simulink model "Battery_droop_control_4"  (R2022a)
settings: Solver=ode23tb  StartTime=0.0  StopTime=1  RelTol=1e-3  EnableMultiTasking=on
values from neighbouring files (symbols this model uses):
  R_power_mode_load_change = zeros(1, length(load_percent_list))    [Battery_charge_discharge_FSBB_param_init.m]
  R_voltage_mode_load_change = zeros(1, length(load_percent_list))    [Battery_charge_discharge_FSBB_param_init.m]
  time_step = 1 / wave_freq    (= 2.22222222222e-05)    [Battery_charge_discharge_FSBB_param_init.m]
undefined symbols (not defined in the file or in its folder): Ion, Lithium
libraries: spsSeriesRLCBranchLib x27, spsTriangleGeneratorLib x16, slpidlib x14, spsCurrentMeasurementLib x9, spsIGBTDiodeLib x8, spsIdealSwitchLib x8, spsVoltageMeasurementLib x8, simulink x4, spsBatteryLib x3, spsControlledVoltageSourceLib x3, eeGeneralControl x2, spspowerguiLib x1
(part 3 of 4)

== system Battery_droop_control_4/InitSystem ==

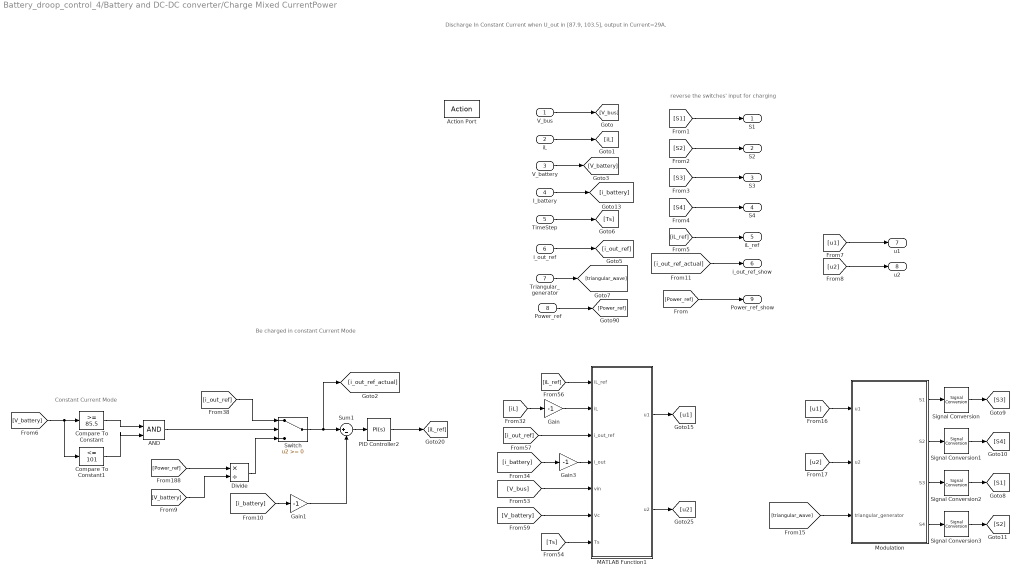
== system Battery_droop_control_4/Battery and DC-DC converter/Charge Mixed CurrentPower ==
  note: Discharge In Constant Current
      | when U_out in [87.9, 103.5], output in Current=29A.
  note: reverse the switches' input for charging
  note: Be charged in constant Current Mode
  note: Constant Current Mode
  V_bus : Inport
  iL : Inport  Port=2
  V_battery : Inport  Port=3
  I_battery : Inport  Port=4
  TimeStep : Inport  Port=5
  i_out_ref : Inport  Port=6
  Triangular_generator : Inport  Port=7
  Power_ref : Inport  Port=8
  Action Port : ActionPort  ActionPortLabel=elseif(u1 == 0 & (u3>=85.5 & u3 <= 116.15))
  AND : Logic  IconShape=distinctive  AllPortsSameDT=off  OutDataTypeStr=boolean
  Compare To Constant : simulink/Logic and Bit Operations/Compare To Constant  relop=>=  const=85.5  OutDataTypeStr=boolean
  Compare To Constant1 : simulink/Logic and Bit Operations/Compare To Constant  relop=<=  const=101  OutDataTypeStr=boolean
  Divide : Product  Inputs=*/
  Gain : Gain  Gain=-1
  Gain1 : Gain  Gain=-1
  Gain3 : Gain  Gain=-1
  MATLAB Function1 : MATLAB Function  TreatAsAtomicUnit=on
  Modulation : Subsystem
  PID Controller2 : slpidlib/PID Controller  Controller=PI  Form=Parallel  TimeDomain=Continuous-time  UseExternalTs=off  SampleTime=-1  IntegratorMethod=Forward Euler  FilterMethod=Forward Euler  ControllerParametersSource=internal  P=15/3  I=1000  UseKiTs=on  D=0  N=100  UseFilter=on  TunerSelectOption=Transfer Function Based (PID Tuner App)  InitialConditionSource=internal  InitialConditionForIntegrator=0  InitialConditionForFilter=0  DifferentiatorICPrevScaledInput=0  ExternalReset=none  TrackingMode=off  Kt=1  LimitOutput=on  SatLimitsSource=internal  UpperSaturationLimit=50  LowerSaturationLimit=-10  LinearizeAsGain=on  AntiWindupMode=clamping  Kb=1  POutMin=[]  POutMax=[]  IOutMin=[]  IOutMax=[]  DOutMin=[]  DOutMax=[]  NOutMin=[]  NOutMax=[]  SumOutMin=[]  SumOutMax=[]  SaturationOutMin=[]  SaturationOutMax=[]  PParamMin=[]  PParamMax=[]  IParamMin=[]  IParamMax=[]  DParamMin=[]  DParamMax=[]  NParamMin=[]  NParamMax=[]  KbParamMin=[]  KbParamMax=[]  KtParamMin=[]  KtParamMax=[]  KbOutMin=[]  KbOutMax=[]  KtOutMin=[]  KtOutMax=[]  IntegratorOutMin=[]  IntegratorOutMax=[]  FilterOutMin=[]  FilterOutMax=[]  SumI1OutMin=[]  SumI1OutMax=[]  SumI2OutMin=[]  SumI2OutMax=[]  SumI3OutMin=[]  SumI3OutMax=[]  SumI4OutMin=[]  SumI4OutMax=[]  SumDOutMin=[]  SumDOutMax=[]  DifferentiatorOutMin=[]  DifferentiatorOutMax=[]  FilterDiffOutCoefMin=[]  FilterDiffOutCoefMax=[]  ReciprocalOutMin=[]  ReciprocalOutMax=[]  SumDenOutMin=[]  SumDenOutMax=[]  SumNumOutMin=[]  SumNumOutMax=[]  DivideOutMin=[]  DivideOutMax=[]  UdiffTsProdOutMin=[]  UdiffTsProdOutMax=[]  NTsProdOutMin=[]  NTsProdOutMax=[]  UintegralTsProdOutMin=[]  UintegralTsProdOutMax=[]  UngainTsProdOutMin=[]  UngainTsProdOutMax=[]  IntegratorContinuousStateAttributes=''  IntegratorStateMustResolveToSignalObject=off  IntegratorRTWStateStorageClass=Auto  FilterContinuousStateAttributes=''  FilterStateMustResolveToSignalObject=off  FilterRTWStateStorageClass=Auto  ParallelPVariant=InternalParameters  IdealPVariant=Disabled  IVariant=InternalParameters  DVariant=Disabled  IntegratorVariant=Continuous  SatVariant=Enabled  AWVariant=ContClampingParallel  PCopyVariant=Disabled  TRVariant=Disabled  FdbkBlocksVariant=Forward  IdealPFdbkVariant=Disabled  SatFdbkVariant=Disabled  DerivativeFilterVariant=Disabled  NVariant=Disabled  NCopyVariant=Disabled_SignalSpec  FilterICVariant=Disabled  IntegratorICVariant=InternalICs  ExternalResetVariant=Disabled  TRSumVariant=Passthrough  SumFdbkVariant=Disabled  SumVariant=Sum_PI  TsampFilterVariant=InternalTs  TsampNgainVariant=Passthrough  TsampIntegralVariant=Passthrough  ExternalSaturationOutDataTypeStr=Inherit: Same as second input  aMode=0
  Signal Conversion{,1..3} (4 alike) : SignalConversion  OverrideOpt=off
  Sum1 : Sum  Inputs=|+-
  Switch : Switch  SaturateOnIntegerOverflow=off  InputSameDT=off
  S1 : Outport
  S2 : Outport  Port=2
  S3 : Outport  Port=3
  S4 : Outport  Port=4
  iL_ref : Outport  Port=5
  i_out_ref_show : Outport  Port=6
  u1 : Outport  Port=7
  u2 : Outport  Port=8
  Power_ref_show : Outport  Port=9
  wires:
  Modulation/2(S2) -> Signal Conversion1/1
  Modulation/1(S1) -> Signal Conversion/1
  Modulation/3(S3) -> Signal Conversion2/1
  [u1] -> Modulation/1(u1)
  [u2] -> Modulation/2(u2)
  Modulation/4(S4) -> Signal Conversion3/1
  V_bus/1 -> [V_bus]
  iL/1 -> [iL]
  V_battery/1 -> [V_battery]
  I_battery/1 -> [i_battery]
  TimeStep/1 -> [Ts]
  i_out_ref/1 -> [i_out_ref]
  [iL_ref] -> iL_ref/1
  [i_out_ref_actual] -> i_out_ref_show/1
  [u2] -> u2/1
  [u1] -> u1/1
  [triangular_wave] -> Modulation/3(triangular_generator)
  Triangular_generator/1 -> [triangular_wave]
  [S1] -> S1/1
  [S3] -> S3/1
  [S4] -> S4/1
  [S2] -> S2/1
  [iL_ref] -> MATLAB Function1/1(iL_ref)
  [V_battery] -> MATLAB Function1/6(Vc)
  [V_bus] -> MATLAB Function1/5(vin)
  Gain/1 -> MATLAB Function1/2(iL)
  [Ts] -> MATLAB Function1/7(Ts)
  [iL] -> Gain/1
  [i_out_ref] -> MATLAB Function1/3(i_out_ref)
  MATLAB Function1/2(u2) -> [u2]
  Gain3/1 -> MATLAB Function1/4(i_out)
  [i_battery] -> Gain3/1
  MATLAB Function1/1(u1) -> [u1]
  Signal Conversion/1 -> [S3]
  Signal Conversion1/1 -> [S4]
  Signal Conversion2/1 -> [S1]
  Signal Conversion3/1 -> [S2]
  Power_ref/1 -> [Power_ref]
  [Power_ref] -> Power_ref_show/1
  Divide/1 -> Switch/3
  [V_battery] -> Divide/2
  Compare To Constant/1 -> AND/1
  [i_out_ref] -> Switch/1
  [Power_ref] -> Divide/1
  PID Controller2/1 -> [iL_ref]
  [V_battery] -> Compare To Constant1/1, Compare To Constant/1
  Switch/1 -> [i_out_ref_actual], Sum1/1
  Compare To Constant1/1 -> AND/2
  Sum1/1 -> PID Controller2/1
  AND/1 -> Switch/2
  [i_battery] -> Gain1/1
  Gain1/1 -> Sum1/2

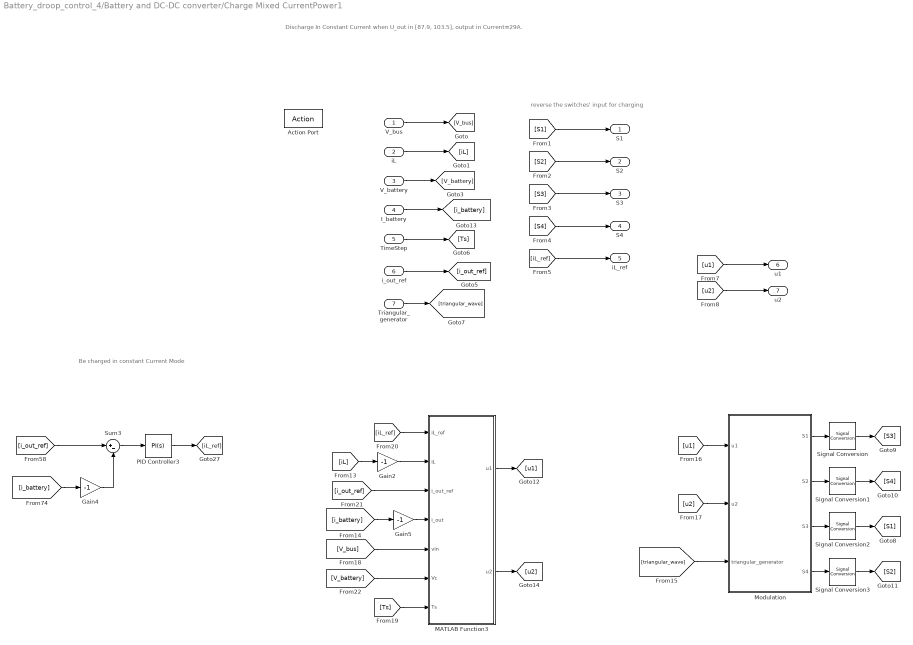
== system Battery_droop_control_4/Battery and DC-DC converter/Charge Mixed CurrentPower1 ==
  note: Discharge In Constant Current
      | when U_out in [87.9, 103.5], output in Current=29A.
  note: reverse the switches' input for charging
  note: Be charged in constant Current Mode
  V_bus : Inport
  iL : Inport  Port=2
  V_battery : Inport  Port=3
  I_battery : Inport  Port=4
  TimeStep : Inport  Port=5
  i_out_ref : Inport  Port=6
  Triangular_generator : Inport  Port=7
  Action Port : ActionPort  ActionPortLabel=elseif(u1 == 0 & u4 < 95)
  Gain2 : Gain  Gain=-1
  Gain4 : Gain  Gain=-1
  Gain5 : Gain  Gain=-1
  MATLAB Function3 : MATLAB Function  TreatAsAtomicUnit=on
  Modulation : Subsystem
  PID Controller3 : slpidlib/PID Controller  Controller=PI  Form=Parallel  TimeDomain=Continuous-time  UseExternalTs=off  SampleTime=-1  IntegratorMethod=Forward Euler  FilterMethod=Forward Euler  ControllerParametersSource=internal  P=6.7500  I=8.1000e+03 * 2  UseKiTs=on  D=0  N=100  UseFilter=on  TunerSelectOption=Transfer Function Based (PID Tuner App)  InitialConditionSource=internal  InitialConditionForIntegrator=0  InitialConditionForFilter=0  DifferentiatorICPrevScaledInput=0  ExternalReset=none  TrackingMode=off  Kt=1  LimitOutput=on  SatLimitsSource=internal  UpperSaturationLimit=50  LowerSaturationLimit=-10  LinearizeAsGain=on  AntiWindupMode=none  Kb=1  POutMin=[]  POutMax=[]  IOutMin=[]  IOutMax=[]  DOutMin=[]  DOutMax=[]  NOutMin=[]  NOutMax=[]  SumOutMin=[]  SumOutMax=[]  SaturationOutMin=[]  SaturationOutMax=[]  PParamMin=[]  PParamMax=[]  IParamMin=[]  IParamMax=[]  DParamMin=[]  DParamMax=[]  NParamMin=[]  NParamMax=[]  KbParamMin=[]  KbParamMax=[]  KtParamMin=[]  KtParamMax=[]  KbOutMin=[]  KbOutMax=[]  KtOutMin=[]  KtOutMax=[]  IntegratorOutMin=[]  IntegratorOutMax=[]  FilterOutMin=[]  FilterOutMax=[]  SumI1OutMin=[]  SumI1OutMax=[]  SumI2OutMin=[]  SumI2OutMax=[]  SumI3OutMin=[]  SumI3OutMax=[]  SumI4OutMin=[]  SumI4OutMax=[]  SumDOutMin=[]  SumDOutMax=[]  DifferentiatorOutMin=[]  DifferentiatorOutMax=[]  FilterDiffOutCoefMin=[]  FilterDiffOutCoefMax=[]  ReciprocalOutMin=[]  ReciprocalOutMax=[]  SumDenOutMin=[]  SumDenOutMax=[]  SumNumOutMin=[]  SumNumOutMax=[]  DivideOutMin=[]  DivideOutMax=[]  UdiffTsProdOutMin=[]  UdiffTsProdOutMax=[]  NTsProdOutMin=[]  NTsProdOutMax=[]  UintegralTsProdOutMin=[]  UintegralTsProdOutMax=[]  UngainTsProdOutMin=[]  UngainTsProdOutMax=[]  IntegratorContinuousStateAttributes=''  IntegratorStateMustResolveToSignalObject=off  IntegratorRTWStateStorageClass=Auto  FilterContinuousStateAttributes=''  FilterStateMustResolveToSignalObject=off  FilterRTWStateStorageClass=Auto  ParallelPVariant=InternalParameters  IdealPVariant=Disabled  IVariant=InternalParameters  DVariant=Disabled  IntegratorVariant=Continuous  SatVariant=Enabled  AWVariant=Passthrough  PCopyVariant=Disabled  TRVariant=Disabled  FdbkBlocksVariant=Forward  IdealPFdbkVariant=Disabled  SatFdbkVariant=Disabled  DerivativeFilterVariant=Disabled  NVariant=Disabled  NCopyVariant=Disabled_SignalSpec  FilterICVariant=Disabled  IntegratorICVariant=InternalICs  ExternalResetVariant=Disabled  TRSumVariant=Passthrough  SumFdbkVariant=Disabled  SumVariant=Sum_PI  TsampFilterVariant=InternalTs  TsampNgainVariant=Passthrough  TsampIntegralVariant=Passthrough  ExternalSaturationOutDataTypeStr=Inherit: Same as second input
  Signal Conversion{,1..3} (4 alike) : SignalConversion  OverrideOpt=off
  Sum3 : Sum  Inputs=|+-
  S1 : Outport
  S2 : Outport  Port=2
  S3 : Outport  Port=3
  S4 : Outport  Port=4
  iL_ref : Outport  Port=5
  u1 : Outport  Port=6
  u2 : Outport  Port=7
  wires:
  Modulation/2(S2) -> Signal Conversion1/1
  Modulation/1(S1) -> Signal Conversion/1
  Modulation/3(S3) -> Signal Conversion2/1
  [u1] -> Modulation/1(u1)
  [u2] -> Modulation/2(u2)
  Modulation/4(S4) -> Signal Conversion3/1
  V_bus/1 -> [V_bus]
  iL/1 -> [iL]
  V_battery/1 -> [V_battery]
  I_battery/1 -> [i_battery]
  TimeStep/1 -> [Ts]
  i_out_ref/1 -> [i_out_ref]
  [iL_ref] -> iL_ref/1
  [u2] -> u2/1
  [u1] -> u1/1
  [triangular_wave] -> Modulation/3(triangular_generator)
  Triangular_generator/1 -> [triangular_wave]
  [S1] -> S1/1
  [S3] -> S3/1
  [S4] -> S4/1
  [S2] -> S2/1
  Signal Conversion/1 -> [S3]
  Signal Conversion1/1 -> [S4]
  Signal Conversion2/1 -> [S1]
  Signal Conversion3/1 -> [S2]
  Gain4/1 -> Sum3/2
  PID Controller3/1 -> [iL_ref]
  Gain5/1 -> MATLAB Function3/4(i_out)
  [iL_ref] -> MATLAB Function3/1(iL_ref)
  MATLAB Function3/1(u1) -> [u1]
  Sum3/1 -> PID Controller3/1
  Gain2/1 -> MATLAB Function3/2(iL)
  [i_battery] -> Gain5/1
  [iL] -> Gain2/1
  [i_out_ref] -> MATLAB Function3/3(i_out_ref)
  [V_battery] -> MATLAB Function3/6(Vc)
  [i_battery] -> Gain4/1
  [i_out_ref] -> Sum3/1
  [V_bus] -> MATLAB Function3/5(vin)
  MATLAB Function3/2(u2) -> [u2]
  [Ts] -> MATLAB Function3/7(Ts)

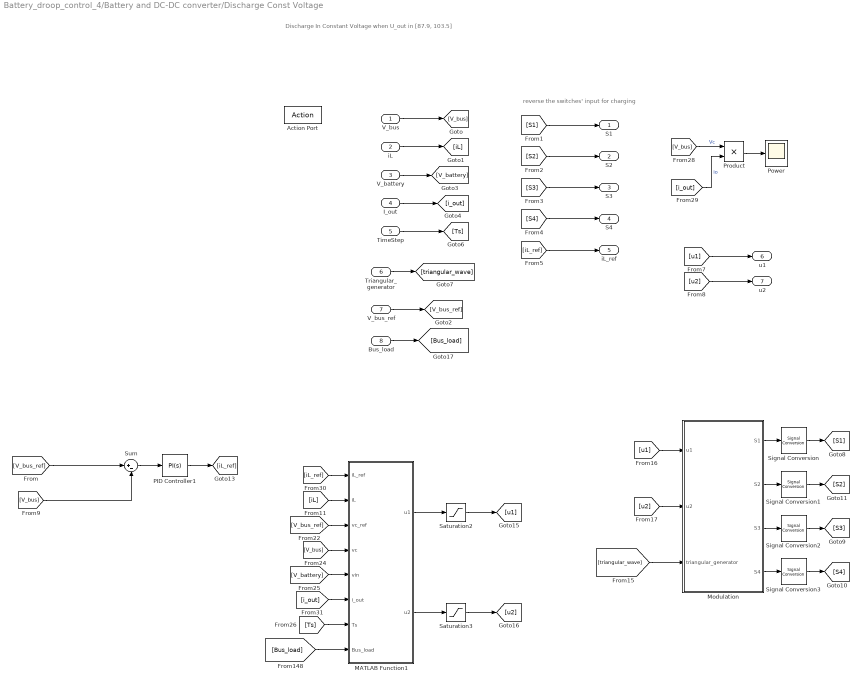
== system Battery_droop_control_4/Battery and DC-DC converter/Discharge Const Voltage ==
  note: Discharge In Constant Voltage
      | when U_out in [87.9, 103.5]
  note: reverse the switches' input for charging
  V_bus : Inport
  iL : Inport  Port=2
  V_battery : Inport  Port=3
  I_out : Inport  Port=4
  TimeStep : Inport  Port=5
  Triangular_generator : Inport  Port=6
  V_bus_ref : Inport  Port=7
  Bus_load : Inport  Port=8
  Action Port : ActionPort  ActionPortLabel="if(u1 == 1  & u4 > 10)"
  MATLAB Function1 : MATLAB Function  TreatAsAtomicUnit=on
  Modulation : Subsystem
  PID Controller1 : slpidlib/PID Controller  Controller=PI  Form=Parallel  TimeDomain=Continuous-time  UseExternalTs=off  SampleTime=-1  IntegratorMethod=Forward Euler  FilterMethod=Forward Euler  ControllerParametersSource=internal  P=45 * 2  I=1.3361e+05 /25  UseKiTs=on  D=0  N=100  UseFilter=on  TunerSelectOption=Frequency Response Based  InitialConditionSource=internal  InitialConditionForIntegrator=0  InitialConditionForFilter=0  DifferentiatorICPrevScaledInput=0  ExternalReset=none  TrackingMode=off  Kt=1  LimitOutput=on  SatLimitsSource=internal  UpperSaturationLimit=50  LowerSaturationLimit=-10  LinearizeAsGain=on  AntiWindupMode=none  Kb=1  POutMin=[]  POutMax=[]  IOutMin=[]  IOutMax=[]  DOutMin=[]  DOutMax=[]  NOutMin=[]  NOutMax=[]  SumOutMin=[]  SumOutMax=[]  SaturationOutMin=[]  SaturationOutMax=[]  PParamMin=[]  PParamMax=[]  IParamMin=[]  IParamMax=[]  DParamMin=[]  DParamMax=[]  NParamMin=[]  NParamMax=[]  KbParamMin=[]  KbParamMax=[]  KtParamMin=[]  KtParamMax=[]  KbOutMin=[]  KbOutMax=[]  KtOutMin=[]  KtOutMax=[]  IntegratorOutMin=[]  IntegratorOutMax=[]  FilterOutMin=[]  FilterOutMax=[]  SumI1OutMin=[]  SumI1OutMax=[]  SumI2OutMin=[]  SumI2OutMax=[]  SumI3OutMin=[]  SumI3OutMax=[]  SumI4OutMin=[]  SumI4OutMax=[]  SumDOutMin=[]  SumDOutMax=[]  DifferentiatorOutMin=[]  DifferentiatorOutMax=[]  FilterDiffOutCoefMin=[]  FilterDiffOutCoefMax=[]  ReciprocalOutMin=[]  ReciprocalOutMax=[]  SumDenOutMin=[]  SumDenOutMax=[]  SumNumOutMin=[]  SumNumOutMax=[]  DivideOutMin=[]  DivideOutMax=[]  UdiffTsProdOutMin=[]  UdiffTsProdOutMax=[]  NTsProdOutMin=[]  NTsProdOutMax=[]  UintegralTsProdOutMin=[]  UintegralTsProdOutMax=[]  UngainTsProdOutMin=[]  UngainTsProdOutMax=[]  IntegratorContinuousStateAttributes=''  IntegratorStateMustResolveToSignalObject=off  IntegratorRTWStateStorageClass=Auto  FilterContinuousStateAttributes=''  FilterStateMustResolveToSignalObject=off  FilterRTWStateStorageClass=Auto  ParallelPVariant=InternalParameters  IdealPVariant=Disabled  IVariant=InternalParameters  DVariant=Disabled  IntegratorVariant=Continuous  SatVariant=Enabled  AWVariant=Passthrough  PCopyVariant=Disabled  TRVariant=Disabled  FdbkBlocksVariant=Forward  IdealPFdbkVariant=Disabled  SatFdbkVariant=Disabled  DerivativeFilterVariant=Disabled  NVariant=Disabled  NCopyVariant=Disabled_SignalSpec  FilterICVariant=Disabled  IntegratorICVariant=InternalICs  ExternalResetVariant=Disabled  TRSumVariant=Passthrough  SumFdbkVariant=Disabled  SumVariant=Sum_PI  TsampFilterVariant=InternalTs  TsampNgainVariant=Passthrough  TsampIntegralVariant=Passthrough  ExternalSaturationOutDataTypeStr=Inherit: Same as second input
  Power : Scope
  Product : Product
  Saturation2 : Saturate  UpperLimit=10  LowerLimit=-10
  Saturation3 : Saturate  UpperLimit=10  LowerLimit=-10  LinearizeAsGain=off
  Signal Conversion{,1..3} (4 alike) : SignalConversion  OverrideOpt=off
  Sum : Sum  Inputs=|+-
  S1 : Outport
  S2 : Outport  Port=2
  S3 : Outport  Port=3
  S4 : Outport  Port=4
  iL_ref : Outport  Port=5
  u1 : Outport  Port=6
  u2 : Outport  Port=7
  wires:
  Modulation/2(S2) -> Signal Conversion1/1
  Modulation/1(S1) -> Signal Conversion/1
  Modulation/3(S3) -> Signal Conversion2/1
  [u1] -> Modulation/1(u1)
  [i_out] -> Product/2  "io"
  [u2] -> Modulation/2(u2)
  [V_bus] -> Product/1  "Vc"
  Product/1 -> Power/1
  Modulation/4(S4) -> Signal Conversion3/1
  V_bus/1 -> [V_bus]
  iL/1 -> [iL]
  V_battery/1 -> [V_battery]
  I_out/1 -> [i_out]
  TimeStep/1 -> [Ts]
  [iL_ref] -> iL_ref/1
  [u2] -> u2/1
  [u1] -> u1/1
  [triangular_wave] -> Modulation/3(triangular_generator)
  Triangular_generator/1 -> [triangular_wave]
  Signal Conversion/1 -> [S1]
  Signal Conversion1/1 -> [S2]
  Signal Conversion2/1 -> [S3]
  Signal Conversion3/1 -> [S4]
  [S1] -> S1/1
  [S3] -> S3/1
  [S4] -> S4/1
  [S2] -> S2/1
  V_bus_ref/1 -> [V_bus_ref]
  PID Controller1/1 -> [iL_ref]
  [V_bus] -> Sum/2
  [V_bus_ref] -> Sum/1
  Sum/1 -> PID Controller1/1
  [Bus_load] -> MATLAB Function1/8(Bus_load)
  MATLAB Function1/2(u2) -> Saturation3/1
  Saturation3/1 -> [u2]
  Saturation2/1 -> [u1]
  MATLAB Function1/1(u1) -> Saturation2/1
  [V_battery] -> MATLAB Function1/5(vin)
  [iL] -> MATLAB Function1/2(iL)
  [iL_ref] -> MATLAB Function1/1(iL_ref)
  [Ts] -> MATLAB Function1/7(Ts)
  [V_bus_ref] -> MATLAB Function1/3(vc_ref)
  [i_out] -> MATLAB Function1/6(i_out)
  [V_bus] -> MATLAB Function1/4(vc)
  Bus_load/1 -> [Bus_load]

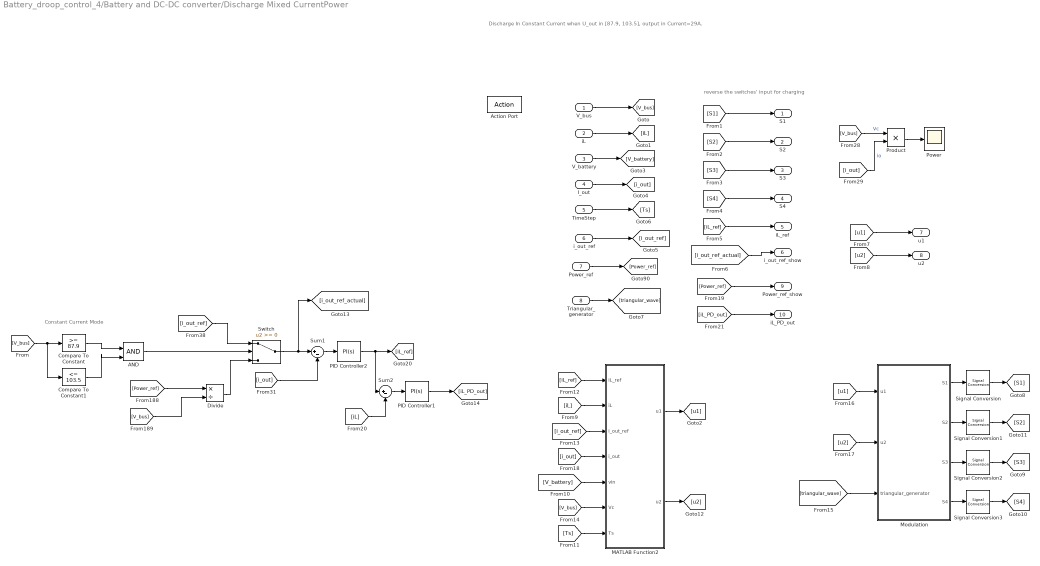
== system Battery_droop_control_4/Battery and DC-DC converter/Discharge Mixed CurrentPower ==
  note: Constant Current Mode
  note: Discharge In Constant Current
      | when U_out in [87.9, 103.5], output in Current=29A.
  note: reverse the switches' input for charging
  V_bus : Inport
  iL : Inport  Port=2
  V_battery : Inport  Port=3
  I_out : Inport  Port=4
  TimeStep : Inport  Port=5
  i_out_ref : Inport  Port=6
  Power_ref : Inport  Port=7
  Triangular_generator : Inport  Port=8
  Action Port : ActionPort  ActionPortLabel=if(u1 == 1 & (u2>=87.9 & u2 <= 119))
  AND : Logic  IconShape=distinctive  AllPortsSameDT=off  OutDataTypeStr=boolean
  Compare To Constant : simulink/Logic and Bit Operations/Compare To Constant  relop=>=  const=87.9  OutDataTypeStr=boolean
  Compare To Constant1 : simulink/Logic and Bit Operations/Compare To Constant  relop=<=  const=103.5  OutDataTypeStr=boolean
  Divide : Product  Inputs=*/
  MATLAB Function2 : MATLAB Function  TreatAsAtomicUnit=on
  Modulation : Subsystem
  PID Controller1 : slpidlib/PID Controller  Controller=PI  Form=Parallel  TimeDomain=Continuous-time  UseExternalTs=off  SampleTime=-1  IntegratorMethod=Forward Euler  FilterMethod=Forward Euler  ControllerParametersSource=internal  P=15/9  I=1000*10  UseKiTs=on  D=0  N=100  UseFilter=on  TunerSelectOption=Transfer Function Based (PID Tuner App)  InitialConditionSource=internal  InitialConditionForIntegrator=0  InitialConditionForFilter=0  DifferentiatorICPrevScaledInput=0  ExternalReset=none  TrackingMode=off  Kt=1  LimitOutput=on  SatLimitsSource=internal  UpperSaturationLimit=50  LowerSaturationLimit=-10  LinearizeAsGain=on  AntiWindupMode=clamping  Kb=1  POutMin=[]  POutMax=[]  IOutMin=[]  IOutMax=[]  DOutMin=[]  DOutMax=[]  NOutMin=[]  NOutMax=[]  SumOutMin=[]  SumOutMax=[]  SaturationOutMin=[]  SaturationOutMax=[]  PParamMin=[]  PParamMax=[]  IParamMin=[]  IParamMax=[]  DParamMin=[]  DParamMax=[]  NParamMin=[]  NParamMax=[]  KbParamMin=[]  KbParamMax=[]  KtParamMin=[]  KtParamMax=[]  KbOutMin=[]  KbOutMax=[]  KtOutMin=[]  KtOutMax=[]  IntegratorOutMin=[]  IntegratorOutMax=[]  FilterOutMin=[]  FilterOutMax=[]  SumI1OutMin=[]  SumI1OutMax=[]  SumI2OutMin=[]  SumI2OutMax=[]  SumI3OutMin=[]  SumI3OutMax=[]  SumI4OutMin=[]  SumI4OutMax=[]  SumDOutMin=[]  SumDOutMax=[]  DifferentiatorOutMin=[]  DifferentiatorOutMax=[]  FilterDiffOutCoefMin=[]  FilterDiffOutCoefMax=[]  ReciprocalOutMin=[]  ReciprocalOutMax=[]  SumDenOutMin=[]  SumDenOutMax=[]  SumNumOutMin=[]  SumNumOutMax=[]  DivideOutMin=[]  DivideOutMax=[]  UdiffTsProdOutMin=[]  UdiffTsProdOutMax=[]  NTsProdOutMin=[]  NTsProdOutMax=[]  UintegralTsProdOutMin=[]  UintegralTsProdOutMax=[]  UngainTsProdOutMin=[]  UngainTsProdOutMax=[]  IntegratorContinuousStateAttributes=''  IntegratorStateMustResolveToSignalObject=off  IntegratorRTWStateStorageClass=Auto  FilterContinuousStateAttributes=''  FilterStateMustResolveToSignalObject=off  FilterRTWStateStorageClass=Auto  ParallelPVariant=InternalParameters  IdealPVariant=Disabled  IVariant=InternalParameters  DVariant=Disabled  IntegratorVariant=Continuous  SatVariant=Enabled  AWVariant=ContClampingParallel  PCopyVariant=Disabled  TRVariant=Disabled  FdbkBlocksVariant=Forward  IdealPFdbkVariant=Disabled  SatFdbkVariant=Disabled  DerivativeFilterVariant=Disabled  NVariant=Disabled  NCopyVariant=Disabled_SignalSpec  FilterICVariant=Disabled  IntegratorICVariant=InternalICs  ExternalResetVariant=Disabled  TRSumVariant=Passthrough  SumFdbkVariant=Disabled  SumVariant=Sum_PI  TsampFilterVariant=InternalTs  TsampNgainVariant=Passthrough  TsampIntegralVariant=Passthrough  ExternalSaturationOutDataTypeStr=Inherit: Same as second input
  PID Controller2 : slpidlib/PID Controller  Controller=PI  Form=Parallel  TimeDomain=Continuous-time  UseExternalTs=off  SampleTime=-1  IntegratorMethod=Forward Euler  FilterMethod=Forward Euler  ControllerParametersSource=internal  P=15/3  I=1000  UseKiTs=on  D=0  N=100  UseFilter=on  TunerSelectOption=Transfer Function Based (PID Tuner App)  InitialConditionSource=internal  InitialConditionForIntegrator=0  InitialConditionForFilter=0  DifferentiatorICPrevScaledInput=0  ExternalReset=none  TrackingMode=off  Kt=1  LimitOutput=on  SatLimitsSource=internal  UpperSaturationLimit=50  LowerSaturationLimit=-10  LinearizeAsGain=on  AntiWindupMode=clamping  Kb=1  POutMin=[]  POutMax=[]  IOutMin=[]  IOutMax=[]  DOutMin=[]  DOutMax=[]  NOutMin=[]  NOutMax=[]  SumOutMin=[]  SumOutMax=[]  SaturationOutMin=[]  SaturationOutMax=[]  PParamMin=[]  PParamMax=[]  IParamMin=[]  IParamMax=[]  DParamMin=[]  DParamMax=[]  NParamMin=[]  NParamMax=[]  KbParamMin=[]  KbParamMax=[]  KtParamMin=[]  KtParamMax=[]  KbOutMin=[]  KbOutMax=[]  KtOutMin=[]  KtOutMax=[]  IntegratorOutMin=[]  IntegratorOutMax=[]  FilterOutMin=[]  FilterOutMax=[]  SumI1OutMin=[]  SumI1OutMax=[]  SumI2OutMin=[]  SumI2OutMax=[]  SumI3OutMin=[]  SumI3OutMax=[]  SumI4OutMin=[]  SumI4OutMax=[]  SumDOutMin=[]  SumDOutMax=[]  DifferentiatorOutMin=[]  DifferentiatorOutMax=[]  FilterDiffOutCoefMin=[]  FilterDiffOutCoefMax=[]  ReciprocalOutMin=[]  ReciprocalOutMax=[]  SumDenOutMin=[]  SumDenOutMax=[]  SumNumOutMin=[]  SumNumOutMax=[]  DivideOutMin=[]  DivideOutMax=[]  UdiffTsProdOutMin=[]  UdiffTsProdOutMax=[]  NTsProdOutMin=[]  NTsProdOutMax=[]  UintegralTsProdOutMin=[]  UintegralTsProdOutMax=[]  UngainTsProdOutMin=[]  UngainTsProdOutMax=[]  IntegratorContinuousStateAttributes=''  IntegratorStateMustResolveToSignalObject=off  IntegratorRTWStateStorageClass=Auto  FilterContinuousStateAttributes=''  FilterStateMustResolveToSignalObject=off  FilterRTWStateStorageClass=Auto  ParallelPVariant=InternalParameters  IdealPVariant=Disabled  IVariant=InternalParameters  DVariant=Disabled  IntegratorVariant=Continuous  SatVariant=Enabled  AWVariant=ContClampingParallel  PCopyVariant=Disabled  TRVariant=Disabled  FdbkBlocksVariant=Forward  IdealPFdbkVariant=Disabled  SatFdbkVariant=Disabled  DerivativeFilterVariant=Disabled  NVariant=Disabled  NCopyVariant=Disabled_SignalSpec  FilterICVariant=Disabled  IntegratorICVariant=InternalICs  ExternalResetVariant=Disabled  TRSumVariant=Passthrough  SumFdbkVariant=Disabled  SumVariant=Sum_PI  TsampFilterVariant=InternalTs  TsampNgainVariant=Passthrough  TsampIntegralVariant=Passthrough  ExternalSaturationOutDataTypeStr=Inherit: Same as second input
  Power : Scope
  Product : Product
  Signal Conversion{,1..3} (4 alike) : SignalConversion  OverrideOpt=off
  Sum1 : Sum  Inputs=|+-
  Sum2 : Sum  Inputs=|+-
  Switch : Switch  SaturateOnIntegerOverflow=off  InputSameDT=off
  S1 : Outport
  S2 : Outport  Port=2
  S3 : Outport  Port=3
  S4 : Outport  Port=4
  iL_ref : Outport  Port=5
  i_out_ref_show : Outport  Port=6
  u1 : Outport  Port=7
  u2 : Outport  Port=8
  Power_ref_show : Outport  Port=9
  iL_PD_out : Outport  Port=10
  wires:
  Modulation/2(S2) -> Signal Conversion1/1
  Modulation/1(S1) -> Signal Conversion/1
  Modulation/3(S3) -> Signal Conversion2/1
  [u1] -> Modulation/1(u1)
  [i_out] -> Product/2  "io"
  [u2] -> Modulation/2(u2)
  [V_bus] -> Product/1  "Vc"
  Product/1 -> Power/1
  Modulation/4(S4) -> Signal Conversion3/1
  V_bus/1 -> [V_bus]
  iL/1 -> [iL]
  V_battery/1 -> [V_battery]
  I_out/1 -> [i_out]
  TimeStep/1 -> [Ts]
  i_out_ref/1 -> [i_out_ref]
  [iL_ref] -> iL_ref/1
  [i_out_ref_actual] -> i_out_ref_show/1
  [u2] -> u2/1
  [u1] -> u1/1
  [triangular_wave] -> Modulation/3(triangular_generator)
  Triangular_generator/1 -> [triangular_wave]
  Signal Conversion/1 -> [S1]
  Signal Conversion1/1 -> [S2]
  Signal Conversion2/1 -> [S3]
  Signal Conversion3/1 -> [S4]
  [i_out] -> Sum1/2
  [S1] -> S1/1
  [S3] -> S3/1
  [S4] -> S4/1
  [S2] -> S2/1
  [i_out] -> MATLAB Function2/4(i_out)
  [i_out_ref] -> MATLAB Function2/3(i_out_ref)
  [V_bus] -> MATLAB Function2/6(Vc)
  [iL] -> MATLAB Function2/2(iL)
  [V_battery] -> MATLAB Function2/5(vin)
  MATLAB Function2/2(u2) -> [u2]
  MATLAB Function2/1(u1) -> [u1]
  [iL_ref] -> MATLAB Function2/1(iL_ref)
  [Ts] -> MATLAB Function2/7(Ts)
  PID Controller2/1 -> Sum2/1, [iL_ref]
  Sum1/1 -> PID Controller2/1
  Switch/1 -> [i_out_ref_actual], Sum1/1
  [i_out_ref] -> Switch/1
  [Power_ref] -> Divide/1
  [V_bus] -> Divide/2
  Divide/1 -> Switch/3
  Power_ref/1 -> [Power_ref]
  [V_bus] -> Compare To Constant1/1, Compare To Constant/1
  Compare To Constant/1 -> AND/1
  Compare To Constant1/1 -> AND/2
  AND/1 -> Switch/2
  [Power_ref] -> Power_ref_show/1
  Sum2/1 -> PID Controller1/1
  [iL] -> Sum2/2
  PID Controller1/1 -> [iL_PD_out]
  [iL_PD_out] -> iL_PD_out/1

== system Battery_droop_control_4/Battery and DC-DC converter/DoNothing1 ==
  Action Port : ActionPort  ActionPortLabel=else
  Constant : Constant
  Terminator : Terminator
  wires:
  Constant/1 -> Terminator/1

== system Battery_droop_control_4/Battery and DC-DC converter/DoNothing2 ==
  Action Port : ActionPort  ActionPortLabel=else
  Constant : Constant
  Output : Outport
  wires:
  Constant/1 -> Output/1

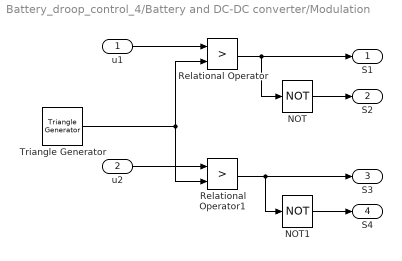
== system Battery_droop_control_4/Battery and DC-DC converter/Modulation ==
  u1 : Inport
  u2 : Inport  Port=2
  NOT : Logic  Operator=NOT  AllPortsSameDT=off  OutDataTypeStr=boolean
  NOT1 : Logic  Operator=NOT  AllPortsSameDT=off  OutDataTypeStr=boolean
  Relational Operator : RelationalOperator  Operator=>  OutDataTypeStr=boolean  RndMeth=Simplest  InputSameDT=off
  Relational Operator1 : RelationalOperator  Operator=>  OutDataTypeStr=boolean  RndMeth=Simplest  InputSameDT=off
  Triangle Generator : spsTriangleGeneratorLib/Triangle Generator  Freq=wave_freq  Phase=0  Ts=0
  S1 : Outport
  S2 : Outport  Port=2
  S3 : Outport  Port=3
  S4 : Outport  Port=4
  wires:
  u1/1 -> Relational Operator/1
  Triangle Generator/1 -> Relational Operator1/2, Relational Operator/2
  u2/1 -> Relational Operator1/1
  Relational Operator/1 -> NOT/1, S1/1
  NOT/1 -> S2/1
  Relational Operator1/1 -> NOT1/1, S3/1
  NOT1/1 -> S4/1

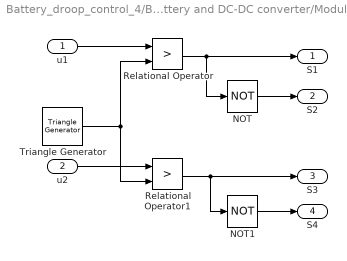
== system Battery_droop_control_4/Battery and DC-DC converter/Modulation1 ==
  u1 : Inport
  u2 : Inport  Port=2
  NOT : Logic  Operator=NOT  AllPortsSameDT=off  OutDataTypeStr=boolean
  NOT1 : Logic  Operator=NOT  AllPortsSameDT=off  OutDataTypeStr=boolean
  Relational Operator : RelationalOperator  Operator=>  OutDataTypeStr=boolean  RndMeth=Simplest  InputSameDT=off
  Relational Operator1 : RelationalOperator  Operator=>  OutDataTypeStr=boolean  RndMeth=Simplest  InputSameDT=off
  Triangle Generator : spsTriangleGeneratorLib/Triangle Generator  Freq=wave_freq  Phase=0  Ts=0
  S1 : Outport
  S2 : Outport  Port=2
  S3 : Outport  Port=3
  S4 : Outport  Port=4
  wires:
  u1/1 -> Relational Operator/1
  Triangle Generator/1 -> Relational Operator1/2, Relational Operator/2
  u2/1 -> Relational Operator1/1
  Relational Operator/1 -> NOT/1, S1/1
  NOT/1 -> S2/1
  Relational Operator1/1 -> NOT1/1, S3/1
  NOT1/1 -> S4/1

== system Battery_droop_control_4/Battery and DC-DC converter/Modulation2 ==
  u1 : Inport
  u2 : Inport  Port=2
  NOT : Logic  Operator=NOT  AllPortsSameDT=off  OutDataTypeStr=boolean
  NOT1 : Logic  Operator=NOT  AllPortsSameDT=off  OutDataTypeStr=boolean
  Relational Operator : RelationalOperator  Operator=>  OutDataTypeStr=boolean  RndMeth=Simplest  InputSameDT=off
  Relational Operator1 : RelationalOperator  Operator=>  OutDataTypeStr=boolean  RndMeth=Simplest  InputSameDT=off
  Triangle Generator : spsTriangleGeneratorLib/Triangle Generator  Freq=wave_freq  Phase=0  Ts=0
  S1 : Outport
  S2 : Outport  Port=2
  S3 : Outport  Port=3
  S4 : Outport  Port=4
  wires:
  u1/1 -> Relational Operator/1
  Triangle Generator/1 -> Relational Operator1/2, Relational Operator/2
  u2/1 -> Relational Operator1/1
  Relational Operator/1 -> NOT/1, S1/1
  NOT/1 -> S2/1
  Relational Operator1/1 -> NOT1/1, S3/1
  NOT1/1 -> S4/1

== system Battery_droop_control_4/Battery and DC-DC converter/Modulation3 ==
  u1 : Inport
  u2 : Inport  Port=2
  NOT : Logic  Operator=NOT  AllPortsSameDT=off  OutDataTypeStr=boolean
  NOT1 : Logic  Operator=NOT  AllPortsSameDT=off  OutDataTypeStr=boolean
  Relational Operator : RelationalOperator  Operator=>  OutDataTypeStr=boolean  RndMeth=Simplest  InputSameDT=off
  Relational Operator1 : RelationalOperator  Operator=>  OutDataTypeStr=boolean  RndMeth=Simplest  InputSameDT=off
  Triangle Generator : spsTriangleGeneratorLib/Triangle Generator  Freq=wave_freq  Phase=0  Ts=0
  S1 : Outport
  S2 : Outport  Port=2
  S3 : Outport  Port=3
  S4 : Outport  Port=4
  wires:
  u1/1 -> Relational Operator/1
  Triangle Generator/1 -> Relational Operator1/2, Relational Operator/2
  u2/1 -> Relational Operator1/1
  Relational Operator/1 -> NOT/1, S1/1
  NOT/1 -> S2/1
  Relational Operator1/1 -> NOT1/1, S3/1
  NOT1/1 -> S4/1

== system Battery_droop_control_4/Battery and DC-DC converter/Modulation4 ==
  u1 : Inport
  u2 : Inport  Port=2
  NOT : Logic  Operator=NOT  AllPortsSameDT=off  OutDataTypeStr=boolean
  NOT1 : Logic  Operator=NOT  AllPortsSameDT=off  OutDataTypeStr=boolean
  Relational Operator : RelationalOperator  Operator=>  OutDataTypeStr=boolean  RndMeth=Simplest  InputSameDT=off
  Relational Operator1 : RelationalOperator  Operator=>  OutDataTypeStr=boolean  RndMeth=Simplest  InputSameDT=off
  Triangle Generator : spsTriangleGeneratorLib/Triangle Generator  Freq=wave_freq  Phase=0  Ts=0
  S1 : Outport
  S2 : Outport  Port=2
  S3 : Outport  Port=3
  S4 : Outport  Port=4
  wires:
  u1/1 -> Relational Operator/1
  Triangle Generator/1 -> Relational Operator1/2, Relational Operator/2
  u2/1 -> Relational Operator1/1
  Relational Operator/1 -> NOT/1, S1/1
  NOT/1 -> S2/1
  Relational Operator1/1 -> NOT1/1, S3/1
  NOT1/1 -> S4/1

== system Battery_droop_control_4/Battery and DC-DC converter/Modulation5 ==
  u1 : Inport
  u2 : Inport  Port=2
  NOT : Logic  Operator=NOT  AllPortsSameDT=off  OutDataTypeStr=boolean
  NOT1 : Logic  Operator=NOT  AllPortsSameDT=off  OutDataTypeStr=boolean
  Relational Operator : RelationalOperator  Operator=>  OutDataTypeStr=boolean  RndMeth=Simplest  InputSameDT=off
  Relational Operator1 : RelationalOperator  Operator=>  OutDataTypeStr=boolean  RndMeth=Simplest  InputSameDT=off
  Triangle Generator : spsTriangleGeneratorLib/Triangle Generator  Freq=wave_freq  Phase=0  Ts=0
  S1 : Outport
  S2 : Outport  Port=2
  S3 : Outport  Port=3
  S4 : Outport  Port=4
  wires:
  u1/1 -> Relational Operator/1
  Triangle Generator/1 -> Relational Operator1/2, Relational Operator/2
  u2/1 -> Relational Operator1/1
  Relational Operator/1 -> NOT/1, S1/1
  NOT/1 -> S2/1
  Relational Operator1/1 -> NOT1/1, S3/1
  NOT1/1 -> S4/1

== system Battery_droop_control_4/Battery and DC-DC converter/Modulation6 ==
  u1 : Inport
  u2 : Inport  Port=2
  NOT : Logic  Operator=NOT  AllPortsSameDT=off  OutDataTypeStr=boolean
  NOT1 : Logic  Operator=NOT  AllPortsSameDT=off  OutDataTypeStr=boolean
  Relational Operator : RelationalOperator  Operator=>  OutDataTypeStr=boolean  RndMeth=Simplest  InputSameDT=off
  Relational Operator1 : RelationalOperator  Operator=>  OutDataTypeStr=boolean  RndMeth=Simplest  InputSameDT=off
  Triangle Generator : spsTriangleGeneratorLib/Triangle Generator  Freq=wave_freq  Phase=0  Ts=0
  S1 : Outport
  S2 : Outport  Port=2
  S3 : Outport  Port=3
  S4 : Outport  Port=4
  wires:
  u1/1 -> Relational Operator/1
  Triangle Generator/1 -> Relational Operator1/2, Relational Operator/2
  u2/1 -> Relational Operator1/1
  Relational Operator/1 -> NOT/1, S1/1
  NOT/1 -> S2/1
  Relational Operator1/1 -> NOT1/1, S3/1
  NOT1/1 -> S4/1

== system Battery_droop_control_4/Battery and DC-DC converter/Modulation7 ==
  u1 : Inport
  u2 : Inport  Port=2
  NOT : Logic  Operator=NOT  AllPortsSameDT=off  OutDataTypeStr=boolean
  NOT1 : Logic  Operator=NOT  AllPortsSameDT=off  OutDataTypeStr=boolean
  Relational Operator : RelationalOperator  Operator=>  OutDataTypeStr=boolean  RndMeth=Simplest  InputSameDT=off
  Relational Operator1 : RelationalOperator  Operator=>  OutDataTypeStr=boolean  RndMeth=Simplest  InputSameDT=off
  Triangle Generator : spsTriangleGeneratorLib/Triangle Generator  Freq=wave_freq  Phase=0  Ts=0
  S1 : Outport
  S2 : Outport  Port=2
  S3 : Outport  Port=3
  S4 : Outport  Port=4
  wires:
  u1/1 -> Relational Operator/1
  Triangle Generator/1 -> Relational Operator1/2, Relational Operator/2
  u2/1 -> Relational Operator1/1
  Relational Operator/1 -> NOT/1, S1/1
  NOT/1 -> S2/1
  Relational Operator1/1 -> NOT1/1, S3/1
  NOT1/1 -> S4/1

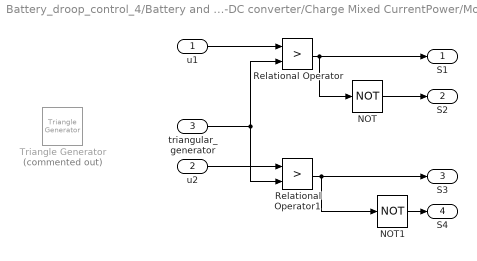
== system Battery_droop_control_4/Battery and DC-DC converter/Charge Mixed CurrentPower/Modulation ==
  u1 : Inport
  u2 : Inport  Port=2
  triangular_generator : Inport  Port=3
  NOT : Logic  Operator=NOT  AllPortsSameDT=off  OutDataTypeStr=boolean
  NOT1 : Logic  Operator=NOT  AllPortsSameDT=off  OutDataTypeStr=boolean
  Relational Operator : RelationalOperator  Operator=>  OutDataTypeStr=boolean  RndMeth=Simplest  InputSameDT=off
  Relational Operator1 : RelationalOperator  Operator=>  OutDataTypeStr=boolean  RndMeth=Simplest  InputSameDT=off
  Triangle Generator : spsTriangleGeneratorLib/Triangle Generator  Commented=on  Freq=wave_freq  Phase=0  Ts=0
  S1 : Outport
  S2 : Outport  Port=2
  S3 : Outport  Port=3
  S4 : Outport  Port=4
  wires:
  u1/1 -> Relational Operator/1
  triangular_generator/1 -> Relational Operator1/2, Relational Operator/2
  u2/1 -> Relational Operator1/1
  NOT1/1 -> S4/1
  Relational Operator/1 -> S1/1, NOT/1
  Relational Operator1/1 -> S3/1, NOT1/1
  NOT/1 -> S2/1

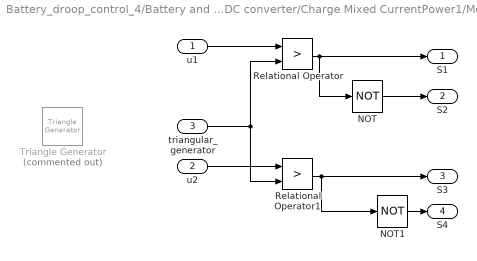
== system Battery_droop_control_4/Battery and DC-DC converter/Charge Mixed CurrentPower1/Modulation ==
  u1 : Inport
  u2 : Inport  Port=2
  triangular_generator : Inport  Port=3
  NOT : Logic  Operator=NOT  AllPortsSameDT=off  OutDataTypeStr=boolean
  NOT1 : Logic  Operator=NOT  AllPortsSameDT=off  OutDataTypeStr=boolean
  Relational Operator : RelationalOperator  Operator=>  OutDataTypeStr=boolean  RndMeth=Simplest  InputSameDT=off
  Relational Operator1 : RelationalOperator  Operator=>  OutDataTypeStr=boolean  RndMeth=Simplest  InputSameDT=off
  Triangle Generator : spsTriangleGeneratorLib/Triangle Generator  Commented=on  Freq=wave_freq  Phase=0  Ts=0
  S1 : Outport
  S2 : Outport  Port=2
  S3 : Outport  Port=3
  S4 : Outport  Port=4
  wires:
  u1/1 -> Relational Operator/1
  triangular_generator/1 -> Relational Operator1/2, Relational Operator/2
  u2/1 -> Relational Operator1/1
  NOT1/1 -> S4/1
  Relational Operator/1 -> S1/1, NOT/1
  Relational Operator1/1 -> S3/1, NOT1/1
  NOT/1 -> S2/1

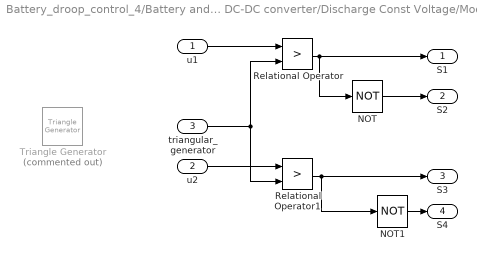
== system Battery_droop_control_4/Battery and DC-DC converter/Discharge Const Voltage/Modulation ==
  u1 : Inport
  u2 : Inport  Port=2
  triangular_generator : Inport  Port=3
  NOT : Logic  Operator=NOT  AllPortsSameDT=off  OutDataTypeStr=boolean
  NOT1 : Logic  Operator=NOT  AllPortsSameDT=off  OutDataTypeStr=boolean
  Relational Operator : RelationalOperator  Operator=>  OutDataTypeStr=boolean  RndMeth=Simplest  InputSameDT=off
  Relational Operator1 : RelationalOperator  Operator=>  OutDataTypeStr=boolean  RndMeth=Simplest  InputSameDT=off
  Triangle Generator : spsTriangleGeneratorLib/Triangle Generator  Commented=on  Freq=wave_freq  Phase=0  Ts=0
  S1 : Outport
  S2 : Outport  Port=2
  S3 : Outport  Port=3
  S4 : Outport  Port=4
  wires:
  u1/1 -> Relational Operator/1
  triangular_generator/1 -> Relational Operator1/2, Relational Operator/2
  u2/1 -> Relational Operator1/1
  NOT1/1 -> S4/1
  Relational Operator/1 -> S1/1, NOT/1
  Relational Operator1/1 -> S3/1, NOT1/1
  NOT/1 -> S2/1

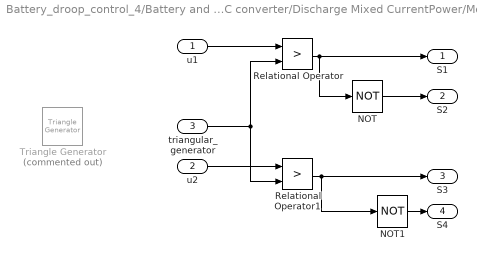
== system Battery_droop_control_4/Battery and DC-DC converter/Discharge Mixed CurrentPower/Modulation ==
  u1 : Inport
  u2 : Inport  Port=2
  triangular_generator : Inport  Port=3
  NOT : Logic  Operator=NOT  AllPortsSameDT=off  OutDataTypeStr=boolean
  NOT1 : Logic  Operator=NOT  AllPortsSameDT=off  OutDataTypeStr=boolean
  Relational Operator : RelationalOperator  Operator=>  OutDataTypeStr=boolean  RndMeth=Simplest  InputSameDT=off
  Relational Operator1 : RelationalOperator  Operator=>  OutDataTypeStr=boolean  RndMeth=Simplest  InputSameDT=off
  Triangle Generator : spsTriangleGeneratorLib/Triangle Generator  Commented=on  Freq=wave_freq  Phase=0  Ts=0
  S1 : Outport
  S2 : Outport  Port=2
  S3 : Outport  Port=3
  S4 : Outport  Port=4
  wires:
  u1/1 -> Relational Operator/1
  triangular_generator/1 -> Relational Operator1/2, Relational Operator/2
  u2/1 -> Relational Operator1/1
  NOT1/1 -> S4/1
  Relational Operator/1 -> S1/1, NOT/1
  Relational Operator1/1 -> S3/1, NOT1/1
  NOT/1 -> S2/1

== matlab function Battery_droop_control_4/Battery and DC-DC converter/MATLAB Function5 ==
  settings: updateMethod=DISCRETE
  data: iL_ref input; u1 output; iL input; i_out_ref input; i_out input; vin input; Vc input; Ts input; u2 output
function [u1, u2] = Passivity_BC(iL_ref, iL,i_out_ref, i_out, vin, Vc, Ts)
% Constant output current Module
% param iL: inductor's current
% param iL_ref: expected value of inductor's current
% param i_out: dcdc output current 
% param i_out_ref
% param vin: input voltage
% param Vc: output voltage
%% system parameters
L = 40e-6;  % Inductance 电感 20uH
L_DMinductor = 2.2e-6;
L = L + L_DMinductor;
RL = 0.004;
C_output = 1440e-6;  % 电容大小

zeta1 = 6;  % dumping gains
zeta2 = 0.08;

% error functions: state variable
x1 = iL - iL_ref;
x2 = i_out - i_out_ref;
persistent iL_ref_old Vc_old;
if isempty(iL_ref_old)
    iL_ref_old = 0;
    Vc_old = 0;
end

diL_ref = (iL_ref - iL_ref_old) / Ts;
dVc_ref = (Vc - Vc_old) / Ts;
%% calculate switching signal: u1,u2
u2 = 1 / iL_ref * (iL_ref - C_output * dVc_ref - i_out_ref + x2*zeta2);
u1 = 1 / vin * (L*diL_ref + RL * iL_ref + Vc * (1 - u2) - x1*zeta1);

iL_ref_old = iL_ref;
Vc_old = Vc;

== matlab function Battery_droop_control_4/Battery and DC-DC converter/Charge Mixed CurrentPower/MATLAB Function1 ==
  settings: updateMethod=DISCRETE
  data: iL_ref input; u1 output; iL input; i_out_ref input; i_out input; vin input; Vc input; Ts input; u2 output
function [u1, u2] = Passivity_BC(iL_ref, iL,i_out_ref, i_out, vin, Vc, Ts)
% Constant output current Module
% param iL: inductor's current
% param iL_ref: expected value of inductor's current
% param i_out: dcdc output current 
% param i_out_ref
% param vin: input voltage
% param Vc: output voltage
%% system parameters
L = 40e-6;  % Inductance 电感 20uH
L_DMinductor = 2.2e-6;
L = L + L_DMinductor;
RL = 0.004;
C_output = 1440e-6;  % 电容大小

zeta1 = 6;  % dumping gains
zeta2 = 0.08;

% error functions: state variable
x1 = iL - iL_ref;
x2 = i_out - i_out_ref;
persistent iL_ref_old Vc_old;
if isempty(iL_ref_old)
    iL_ref_old = 0;
    Vc_old = 0;
end

diL_ref = (iL_ref - iL_ref_old) / Ts;
dVc_ref = (Vc - Vc_old) / Ts;
%% calculate switching signal: u1,u2
u2 = 1 / iL_ref * (iL_ref - C_output * dVc_ref - i_out_ref + x2*zeta2);
u1 = 1 / vin * (L*diL_ref + RL * iL_ref + Vc * (1 - u2) - x1*zeta1);

iL_ref_old = iL_ref;
Vc_old = Vc;

== matlab function Battery_droop_control_4/Battery and DC-DC converter/MATLAB Function4 ==
  settings: updateMethod=DISCRETE
  data: iL_ref input; u1 output; iL input; vc_ref input; vc input; vin input; i_out input; Ts input; u2 output; Bus_load input
function [u1, u2] = Passivity_BC(iL_ref, iL, vc_ref, vc, vin, i_out, Ts, Bus_load)
% Constant output voltage Module
%   param vc_ref: expected
%   param vc: dcdc output voltage
%   param vin: input voltage
%   param io: current in output side
%   param Bus_load:
%% system parameters
L = 40e-6;  % Inductance 电感 20uH
L_DMinductor = 2.5e-6;
L = L + L_DMinductor;
RL = 0.004;
Co = 2440e-6;  % 电容大小

zeta1 = L / RL * 2000;  % dumping gains
zeta2 = Co * 1000; 

% if Bus_load > 1e4
%     zeta2 = 1e-3;
% end


% error functions: state variable
x1 = iL - iL_ref;
x2 = vc - vc_ref;
persistent iL_ref_old vc_ref_old;
if isempty(iL_ref_old)
    iL_ref_old = 0;
    vc_ref_old = 0;
end

diL_ref = (iL_ref - iL_ref_old) / Ts;
dvc_ref = (vc_ref - vc_ref_old) / Ts;
%% calculate switching signal: u1,u2
% u2 denotes S3's state
% u1 denotes S1's state
u2 = 1 / iL_ref * (iL_ref - dvc_ref * Co - i_out + x2*zeta2);
u1 = 1 / vin * (L*diL_ref + RL*iL_ref + vc_ref*(1-u2) - x1*zeta1);
iL_ref_old = iL_ref;
vc_ref_old = vc_ref;

% compensate strategy
S1_duty_cycle = vc_ref / vin;
S4_duty_cycle = 1 - vin / vc_ref;  % vin < vc
S3_duty_cycle = 1- S4_duty_cycle;
PWM_triangular_wave_range = 2;
PWM_triangular_wave_min = -1;
original_u2 = u2;


persistent voltage_surge_max;
if isempty(voltage_surge_max)
    voltage_surge_max = 0;
end

if Bus_load > 1e2
    u2 = S4_duty_cycle;  % need to check
end


% Modify overshoot at initial stage
if vc - vc_ref > 1 %&& (vc - voltage_surge_max > -0.4)
    u2 = 2;
%     u2 = S3_duty_cycle * PWM_triangular_wave_range + PWM_triangular_wave_min;
    if vin - vc_ref > 1
        u1 = (1 - S1_duty_cycle) * PWM_triangular_wave_range + PWM_triangular_wave_min;
    end
end

% BoostMode
if vc_ref -vc > 0.5 % && Bus_load > 1e2
    u2 = S4_duty_cycle;
%     u2 = S3_duty_cycle * PWM_triangular_wave_range + PWM_triangular_wave_min;
    u1 = max(u1, S3_duty_cycle* PWM_triangular_wave_range + PWM_triangular_wave_min);
%     u1 = 2;
end


if abs(i_out) < 5 && abs(vc - vc_ref) < 0.3
    u2 = S4_duty_cycle;
end




% % Boost mode
% if (vc_ref - vin) > 1 && (vc_ref - vc) > 0.5
%     u1 = S1_duty_cycle * PWM_triangular_wave_range + PWM_triangular_wave_min;
% %     u2 = S4_duty_cycle * PWM_triangular_wave_range + PWM_triangular_wave_min;
% end
% 
% % Buck mode
% if vin - vc_ref > 1 && vc - vc_ref > 1
%     u2 = 2;
% %     u1 = S1_duty_cycle * PWM_triangular_wave_range + PWM_triangular_wave_min;
% end

voltage_surge_max = max(vc, voltage_surge_max);

== matlab function Battery_droop_control_4/Battery and DC-DC converter/MATLAB Function6 ==
  settings: updateMethod=DISCRETE
  data: iL_ref input; u1 output; iL input; i_out_ref input; i_out input; vin input; Vc input; Ts input; u2 output
function [u1, u2] = Passivity_BC(iL_ref, iL,i_out_ref, i_out, vin, Vc, Ts)
% Constant output current Module
% param iL: inductor's current
% param iL_ref: expected value of inductor's current
% param i_out: dcdc output current 
% param i_out_ref
% param vin: input voltage
% param Vc: output voltage
%% system parameters
L = 40e-6;  % Inductance 电感 20uH
L_DMinductor = 2.2e-6;
L = L + L_DMinductor;
RL = 0.004;
C_output = 1440e-6;  % 电容大小

zeta1 = 6;  % dumping gains
zeta2 = 0.08;

% error functions: state variable
x1 = iL - iL_ref;
x2 = i_out - i_out_ref;
persistent iL_ref_old Vc_old;
if isempty(iL_ref_old)
    iL_ref_old = 0;
    Vc_old = 0;
end

diL_ref = (iL_ref - iL_ref_old) / Ts;
dVc_ref = (Vc - Vc_old) / Ts;
%% calculate switching signal: u1,u2
u2 = 1 / iL_ref * (iL_ref - C_output * dVc_ref - i_out_ref + x2*zeta2);
u1 = 1 / vin * (L*diL_ref + RL * iL_ref + Vc * (1 - u2) - x1*zeta1);

iL_ref_old = iL_ref;
Vc_old = Vc;

== matlab function Battery_droop_control_4/Battery and DC-DC converter/MATLAB Function1 ==
  settings: updateMethod=DISCRETE
  data: iL_ref input; u1 output; iL input; i_out_ref input; i_out input; vin input; Vc input; Ts input; u2 output
function [u1, u2] = Passivity_BC(iL_ref, iL,i_out_ref, i_out, vin, Vc, Ts)
% Constant output current Module
% param iL: inductor's current
% param iL_ref: expected value of inductor's current
% param i_out: dcdc output current 
% param i_out_ref
% param vin: input voltage
% param Vc: output voltage
%% system parameters
L = 40e-6;  % Inductance 电感 20uH
L_DMinductor = 2.2e-6;
L = L + L_DMinductor;
RL = 0.004;
C_output = 1440e-6;  % 电容大小

% zeta1 = 6*2;  % dumping gains
% zeta2 = 0.08*10;
zeta1 = L / RL * 2000;  % dumping gains
zeta2 = C_output * 1000; 

% error functions: state variable
x1 = iL - iL_ref;
x2 = i_out - i_out_ref;
persistent iL_ref_old Vc_old;
if isempty(iL_ref_old)
    iL_ref_old = 0;
    Vc_old = 0;
end

diL_ref = (iL_ref - iL_ref_old) / Ts;
dVc_ref = (Vc - Vc_old) / Ts;
%% calculate switching signal: u1,u2
u2 = 1 / iL_ref * (iL_ref - C_output * dVc_ref - i_out_ref + x2*zeta2);
u1 = 1 / vin * (L*diL_ref + RL * iL_ref + Vc * (1 - u2) - x1*zeta1);

iL_ref_old = iL_ref;
Vc_old = Vc;

== matlab function Battery_droop_control_4/Battery and DC-DC converter/MATLAB Function7 ==
  settings: updateMethod=DISCRETE
  data: iL_ref input; u1 output; iL input; vc_ref input; vc input; vin input; i_out input; Ts input; u2 output; Bus_load input
function [u1, u2] = Passivity_BC(iL_ref, iL, vc_ref, vc, vin, i_out, Ts, Bus_load)
% Constant output voltage Module
%   param vc_ref: expected
%   param vc: dcdc output voltage
%   param vin: input voltage
%   param io: current in output side
%   param Bus_load:
%% system parameters
L = 40e-6;  % Inductance 电感 20uH
L_DMinductor = 2.2e-6;
L = L + L_DMinductor;
RL = 0.004;
Co = 1440e-6;  % 电容大小

zeta1 = L / RL * 2000;  % dumping gains
zeta2 = Co * 1000; 

% if Bus_load > 1e4
%     zeta2 = 1e-3;
% end


% error functions: state variable
x1 = iL - iL_ref;
x2 = vc - vc_ref;
persistent iL_ref_old vc_ref_old;
if isempty(iL_ref_old)
    iL_ref_old = 0;
    vc_ref_old = 0;
end

diL_ref = (iL_ref - iL_ref_old) / Ts;
dvc_ref = (vc_ref - vc_ref_old) / Ts;
%% calculate switching signal: u1,u2
% u2 denotes S3's state
% u1 denotes S1's state
u2 = 1 / iL_ref * (iL_ref - dvc_ref * Co - i_out + x2*zeta2);
u1 = 1 / vin * (L*diL_ref + RL*iL_ref + vc_ref*(1-u2) - x1*zeta1);
iL_ref_old = iL_ref;
vc_ref_old = vc_ref;

% compensate strategy
S1_duty_cycle = vc_ref / vin;
S4_duty_cycle = 1 - vin / vc_ref;  % vin < vc
S3_duty_cycle = 1- S4_duty_cycle;
PWM_triangular_wave_range = 2;
PWM_triangular_wave_min = -1;
original_u2 = u2;


persistent voltage_surge_max;
if isempty(voltage_surge_max)
    voltage_surge_max = 0;
end

if Bus_load > 1e2
    u2 = S4_duty_cycle;  % need to check
end

% if Bus_load > 1e2 && abs(vc - vc_ref) < 0.2
%     u2 = 0.5 * PWM_triangular_wave_range + PWM_triangular_wave_min;
%     u1 = 0.5 * PWM_triangular_wave_range + PWM_triangular_wave_min;
% end

if vc - vc_ref > 1 && (vc - voltage_surge_max > -0.4)
%     u2 = 2;
    u2 = S3_duty_cycle * PWM_triangular_wave_range + PWM_triangular_wave_min;
end
if vc - vc_ref > 1 && vin - vc_ref > 1
    u1 = (1 - S1_duty_cycle) * PWM_triangular_wave_range + PWM_triangular_wave_min;
end

% solve buck-boost mode: sudden u2=1, keep bucking
if vc_ref -vc > 0.2 && Bus_load > 1e2
    % In buck-boost mode, start boost when vc starts to drop > 0.3V
    u2 = S4_duty_cycle;
    u1 = max(u1, S3_duty_cycle* PWM_triangular_wave_range + PWM_triangular_wave_min);
end

% % Boost mode
% if (vc_ref - vin) > 1 && (vc_ref - vc) > 0.5
%     u1 = S1_duty_cycle * PWM_triangular_wave_range + PWM_triangular_wave_min;
% %     u2 = S4_duty_cycle * PWM_triangular_wave_range + PWM_triangular_wave_min;
% end
% 
% % Buck mode
% if vin - vc_ref > 1 && vc - vc_ref > 1
%     u2 = 2;
% %     u1 = S1_duty_cycle * PWM_triangular_wave_range + PWM_triangular_wave_min;
% end

voltage_surge_max = max(vc, voltage_surge_max);

== matlab function Battery_droop_control_4/Battery and DC-DC converter/Charge Mixed CurrentPower1/MATLAB Function3 ==
  settings: updateMethod=DISCRETE
  data: iL_ref input; u1 output; iL input; i_out_ref input; i_out input; vin input; Vc input; Ts input; u2 output
function [u1, u2] = Passivity_BC(iL_ref, iL,i_out_ref, i_out, vin, Vc, Ts)
% Constant output current Module
% param iL: inductor's current
% param iL_ref: expected value of inductor's current
% param i_out: dcdc output current 
% param i_out_ref
% param vin: input voltage
% param Vc: output voltage
%% system parameters
L = 40e-6;  % Inductance 电感 20uH
L_DMinductor = 2.2e-6;
L = L + L_DMinductor;
RL = 0.004;
C_output = 1440e-6;  % 电容大小

% zeta1 = 6 * 2;  % dumping gains
% zeta2 = 0.08 * 10;
zeta1 = L / RL * 2000;  % dumping gains
zeta2 = C_output * 1000; 

% error functions: state variable
x1 = iL - iL_ref;
x2 = i_out - i_out_ref;
persistent iL_ref_old Vc_old;
if isempty(iL_ref_old)
    iL_ref_old = 0;
    Vc_old = 0;
end

diL_ref = (iL_ref - iL_ref_old) / Ts;
dVc_ref = (Vc - Vc_old) / Ts;
%% calculate switching signal: u1,u2
u2 = 1 / iL_ref * (iL_ref - C_output * dVc_ref - i_out_ref + x2*zeta2);
u1 = 1 / vin * (L*diL_ref + RL * iL_ref + Vc * (1 - u2) - x1*zeta1);

iL_ref_old = iL_ref;
Vc_old = Vc;
